simulink model "B2B_MMC"  (R2018b)
settings: Solver=ode8  StartTime=0.0  StopTime=inf  FixedStep=10e-5  RelTol=1e-3
InitFcn:
  | Cd=100e-6;
  | Csm=3.3e-3;
  | L=4e-3;
  | R=0.1;
  | m=1;
  | N=9;
  | Nminus=N-1;
  | 
  | 
  | grid.vll_rms=10e3;
  | grid.f=50;
  | w=2*pi*grid.f;
  | grid.phase=0;
  | grid.va_peak=sqrt(2/3)*grid.vll_rms;
  | 
  | vd_ref=1.05*2*sqrt(2/3)*grid.vll_rms/m; % dc link voltage in pu
  | vsp_max=0.5*m*vd_ref; %phase voltage at phi=0
  | is_max=907;
  | Smax=3*grid.va_peak*is_max/2;
  | 
  | 
  | SCR= 100;  % INPUT SCR of grid at PCC = Ssc_grid/S_rated
  | %Calculated Grid impedance parameters
  | grid.L=grid.va_peak/(w*SCR*is_max); %Calculate Lg out of SRC and neglecting Rg
  | grid.R= w*grid.L/10;        % assume Rg = 10% of Xg [ohm];
  | grid.enable=1;
  | 
  | 
  | 
  | mmc1.load_percent=100;
  | mmc1.load_pf=0.9;
  | 
  | mmc2.load_percent=100;
  | mmc2.load_pf=0.9;
  | 
  | 
  | 
  | mmc1.occ_alpha = 2000;      % INPUT Desired BW output control test converter [rad/s]
  | mmc1.occ_alpha1 = 50;       % INPUT Desired BW of the resonant integrator [rad/s]
  | mmc1.occ_alpha_f = 1000;       % INPUT Desire BW of the VFF [rad/s]
  | 
  | mmc2.occ_alpha = 2000;      % INPUT Desired BW output control test converter [rad/s]
  | mmc2.occ_alpha1 = 50;       % INPUT Desired BW of the resonant integrator [rad/s}
  | mmc2.occ_alpha_f = 1000;       % INPUT Desire BW of the VFF [rad/s
  | 
  | 
  | mmc1.ccc_enable= 1; %INPUT enable ic controller
  | mmc1.ccc_time_enable= 0; %time when circ current control kicks in [s]
  | mmc1.ccc_alpha_cr= 30;  % INPUT BW of LPF for circ current to get the reference (dc value)[rad/s]
  | mmc1.ccc_Ra        = 10;       % INPUT Proportional gain of circ current control (R << Ra < Kp)
  | mmc1.ccc_alpha2 = 200;      % INPUT BW for circulating current test converter  (alpha_c < wgrid)[rad/s]
  | 
  | mmc2.ccc_enable= 1; %INPUT enable ic controller
  | mmc2.ccc_time_enable= 0; %time when circ current control kicks in [s]
  | mmc2.ccc_alpha_cr= 30;  % INPUT BW of LPF for circ current to get the reference (dc value)[rad/s]
  | mmc2.ccc_Ra        = 10;       % INPUT Proportional gain of circ current control (R << Ra < Kp)
  | mmc2.ccc_alpha2 = 200;      % INPUT BW for circulating current test converter  (alpha_c < wgrid)[rad/s]
  | 
  | 
  | mmc1.aec_enable_W= 1; %INPUT enable arm energy controller (Wsum and Wdelta)) at time_W_ctrl
  | ... (+31 lines)
libraries: powerlib x90, powerlib_meascontrol x10, rtlab x1, rtio_opalrt_op5142ex1 x1
(part 3 of 3)

== system B2B_MMC/SM_MMC/MMC2/Control Box MMC2/Controllers/Circulating Current and Arm Energy Controller/arm energy controller /Wsum  Controller ==
  Kp_Wsum : Gain  Gain=aec.Kp_Wsum
  Mux : Mux  Inputs=2
  Mux1 : Mux  Inputs=3
  Product1 : Product
  Ripple Pass (leg a) : Subsystem
  Ripple Pass (leg b) : Subsystem
  Ripple Pass (leg c) : Subsystem
  Scope7 : Scope
  Step : Step  Time=aec.time_WsumRef_step  Before=1  After=1+aec.WsumRefStep*aec.enable_Wsum_step  SampleTime=0
  Sum6 : Sum  Inputs=+-
  "Wsum* " : Constant  Value=WsumRef
  icWsum* : Outport
  wires:
  Mux1/1 -> Sum6/2, Mux/2
  Sum6/1 -> Kp_Wsum/1
  Step/1 -> Product1/2
  Product1/1 -> Mux/1, Sum6/1
  "Wsum* "/1 -> Product1/1
  Kp_Wsum/1 -> icWsum*/1
  Mux/1 -> Scope7/1
  Ripple Pass (leg b)/1(Out1) -> Mux1/2
  Ripple Pass (leg a)/1(Out1) -> Mux1/1
  Ripple Pass (leg c)/1(Out1) -> Mux1/3
  [vc_ua] -> Ripple Pass (leg a)/1(vc_ua)
  [vc_la] -> Ripple Pass (leg a)/2(vc_la)
  [vc_lb] -> Ripple Pass (leg b)/2(vc_lb)
  [vc_ub] -> Ripple Pass (leg b)/1(vc_ub)
  [vc_lc] -> Ripple Pass (leg c)/2(vc_lc)
  [vc_uc] -> Ripple Pass (leg c)/1(vc_uc)

== system B2B_MMC/SM_MMC/MMC2/Control Box MMC2/Controllers/Circulating Current and Arm Energy Controller/ic controller/SOGI1 ==
  In : Inport
  wo : Inport  Port=2
  RST : Inport  Port=3
  Divide : Product  Inputs=**
  Divide1 : Product  Inputs=**
  Divide2 : Product  Inputs=*/
  Integrator : Integrator  ExternalReset=level
  Integrator1 : Integrator  ExternalReset=level
  Sum3 : Sum  Inputs=|+-
  Out : Outport
  wires:
  Divide1/1 -> Sum3/2
  Divide/1 -> Integrator/1
  Sum3/1 -> Divide/1
  Integrator1/1 -> Divide1/2
  In/1 -> Sum3/1
  Divide2/1 -> Out/1
  RST/1 -> Integrator/2, Integrator1/2
  wo/1 -> Divide2/2, Divide1/1, Divide/2
  Integrator/1 -> Divide2/1, Integrator1/1

== system B2B_MMC/SM_MMC/MMC2/Control Box MMC2/Controllers/Circulating Current and Arm Energy Controller/ic controller/SOGI2 ==
  In : Inport
  wo : Inport  Port=2
  RST : Inport  Port=3
  Divide : Product  Inputs=**
  Divide1 : Product  Inputs=**
  Divide2 : Product  Inputs=*/
  Integrator : Integrator  ExternalReset=level  LimitOutput=on  UpperSaturationLimit=is_max  LowerSaturationLimit=-is_max
  Integrator1 : Integrator  ExternalReset=level  LimitOutput=on  UpperSaturationLimit=is_max  LowerSaturationLimit=-is_max
  Sum3 : Sum  Inputs=|+-
  Out : Outport
  wires:
  Integrator/1 -> Divide2/1, Integrator1/1
  wo/1 -> Divide/2, Divide1/1, Divide2/2
  RST/1 -> Integrator/2, Integrator1/2
  Divide2/1 -> Out/1
  In/1 -> Sum3/1
  Integrator1/1 -> Divide1/2
  Sum3/1 -> Divide/1
  Divide/1 -> Integrator/1
  Divide1/1 -> Sum3/2

== system B2B_MMC/SM_MMC/MMC2/Control Box MMC2/Controllers/PR Output Current Controller/Subsystem/PR ==
  note: SOGI continuous=sw/(s2+w2)
  In : Inport
  w0 : Inport  Port=2
  Gain3 : Gain  Gain=occ.K1
  SOGI : Subsystem
  Step : Step  Time=0.0001  Before=1  After=0  SampleTime=0
  Out : Outport
  wires:
  Gain3/1 -> Out/1
  In/1 -> SOGI/1(In)
  w0/1 -> SOGI/2(wo)
  [occRST] -> SOGI/3(RST)
  SOGI/1(Out) -> Gain3/1
  Step/1 -> [occRST]

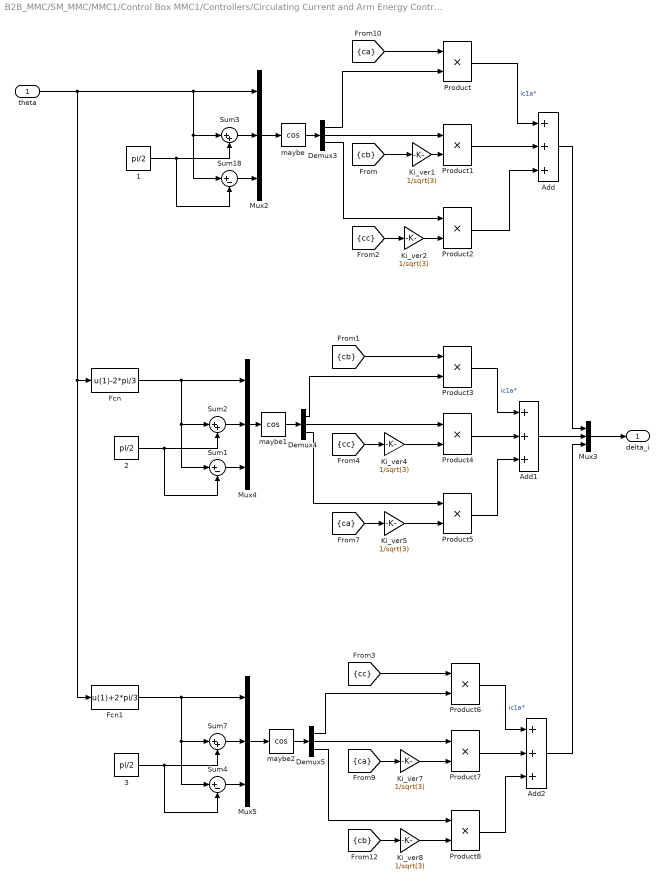
== system B2B_MMC/SM_MMC/MMC1/Control Box MMC1/Controllers/Circulating Current and Arm Energy Controller/arm energy controller /Wdelta  Controller/correction ==
  theta : Inport
  "  1" : Constant  Value=pi/2
  "  2" : Constant  Value=pi/2
  "  3" : Constant  Value=pi/2
  Add : Sum  Inputs=+++
  Add1 : Sum  Inputs=+++
  Add2 : Sum  Inputs=+++
  Demux3 : Demux  Outputs=3
  Demux4 : Demux  Outputs=3
  Demux5 : Demux  Outputs=3
  Fcn : Fcn  Expr=u(1)-2*pi/3
  Fcn1 : Fcn  Expr=u(1)+2*pi/3
  Ki_ver{1..2,4..5,7..8} (6 alike) : Gain  Gain=1/sqrt(3)
  Mux{2..5} (4 alike) : Mux  Inputs=3
  Product{,1..8} (9 alike) : Product
  Sum1 : Sum  Inputs=|+-
  Sum18 : Sum  Inputs=|+-
  Sum2 : Sum  Inputs=|++
  Sum3 : Sum  Inputs=|++
  Sum4 : Sum  Inputs=|+-
  Sum7 : Sum  Inputs=|++
  maybe : Trigonometry  Operator=cos
  maybe1 : Trigonometry  Operator=cos
  maybe2 : Trigonometry  Operator=cos
  delta_i : Outport
  wires:
  Demux4/2 -> Product4/1
  Demux4/3 -> Product5/1
  [ca] -> Product/1
  [ca] -> Ki_ver7/1
  Sum4/1 -> Mux5/3
  Demux4/1 -> Product3/2
  Mux4/1 -> maybe1/1
  Add/1 -> Mux3/1
  Sum3/1 -> Mux2/2
  Ki_ver7/1 -> Product7/2
  Sum7/1 -> Mux5/2
  [cb] -> Ki_ver1/1
  Product1/1 -> Add/2
  Add2/1 -> Mux3/3
  Product5/1 -> Add1/3
  Product8/1 -> Add2/3
  Product3/1 -> Add1/1  "ic1a*"
  Sum18/1 -> Mux2/3
  Add1/1 -> Mux3/2
  "  2"/1 -> Sum1/2, Sum2/2
  Mux5/1 -> maybe2/1
  Demux5/3 -> Product8/1
  Ki_ver4/1 -> Product4/2
  Demux3/1 -> Product/2
  theta/1 -> Mux2/1, Sum3/1, Sum18/1, Fcn/1, Fcn1/1
  maybe1/1 -> Demux4/1
  [cc] -> Ki_ver4/1
  Product7/1 -> Add2/2
  maybe2/1 -> Demux5/1
  Sum2/1 -> Mux4/2
  Demux5/2 -> Product7/1
  Ki_ver5/1 -> Product5/2
  Ki_ver1/1 -> Product1/2
  [cb] -> Product3/1
  Demux5/1 -> Product6/2
  Product/1 -> Add/1  "ic1a*"
  [cb] -> Ki_ver8/1
  maybe/1 -> Demux3/1
  "  3"/1 -> Sum7/2, Sum4/2
  Sum1/1 -> Mux4/3
  Product4/1 -> Add1/2
  Ki_ver2/1 -> Product2/2
  Product2/1 -> Add/3
  [cc] -> Ki_ver2/1
  Ki_ver8/1 -> Product8/2
  "  1"/1 -> Sum3/2, Sum18/2
  Demux3/2 -> Product1/1
  Fcn1/1 -> Mux5/1, Sum7/1, Sum4/1
  Demux3/3 -> Product2/1
  Fcn/1 -> Sum1/1, Sum2/1, Mux4/1
  [ca] -> Ki_ver5/1
  Product6/1 -> Add2/1  "ic1a*"
  Mux2/1 -> maybe/1
  Mux3/1 -> delta_i/1
  [cc] -> Product6/1

== system B2B_MMC/SM_MMC/MMC1/Control Box MMC1/Controllers/Circulating Current and Arm Energy Controller/arm energy controller /Wdelta  Controller/ripple pass (leg a) ==
  vc_ua : Inport
  vc_la : Inport  Port=2
  BandStop @100Hz_10kHz : TransferFcn  Numerator=[1 0 2*w*2*w]  Denominator=[1 2*2*w 2*w*2*w]
  BandStop @50Hz_10kHz1 : TransferFcn  Numerator=[1 0 w*w]  Denominator=[1 2*w w*w]
  Gain : Gain  Gain=Csm/2/N
  Math Function : Math  Operator=square  SaturateOnIntegerOverflow=on
  Math Function1 : Math  Operator=square  SaturateOnIntegerOverflow=on
  Sum : Sum  Inputs=|+-
  Sum of Elements : Sum  Inputs=+
  Sum of Elements1 : Sum  Inputs=+
  Out1 : Outport
  wires:
  BandStop @100Hz_10kHz/1 -> Out1/1
  Math Function1/1 -> Sum/2
  Gain/1 -> BandStop @50Hz_10kHz1/1
  Math Function/1 -> Sum/1
  BandStop @50Hz_10kHz1/1 -> BandStop @100Hz_10kHz/1
  Sum/1 -> Gain/1
  Sum of Elements/1 -> Math Function/1
  vc_ua/1 -> Sum of Elements/1
  Sum of Elements1/1 -> Math Function1/1
  vc_la/1 -> Sum of Elements1/1

== system B2B_MMC/SM_MMC/MMC1/Control Box MMC1/Controllers/Circulating Current and Arm Energy Controller/arm energy controller /Wdelta  Controller/ripple pass (leg b) ==
  vc_ub : Inport
  vc_lb : Inport  Port=2
  BandStop @100Hz_10kHz : TransferFcn  Numerator=[1 0 2*w*2*w]  Denominator=[1 2*2*w 2*w*2*w]
  BandStop @50Hz_10kHz1 : TransferFcn  Numerator=[1 0 w*w]  Denominator=[1 2*w w*w]
  Gain : Gain  Gain=Csm/2/N
  Math Function : Math  Operator=square  SaturateOnIntegerOverflow=on
  Math Function1 : Math  Operator=square  SaturateOnIntegerOverflow=on
  Sum : Sum  Inputs=|+-
  Sum of Elements : Sum  Inputs=+
  Sum of Elements1 : Sum  Inputs=+
  Out1 : Outport
  wires:
  BandStop @100Hz_10kHz/1 -> Out1/1
  Math Function1/1 -> Sum/2
  Gain/1 -> BandStop @50Hz_10kHz1/1
  Math Function/1 -> Sum/1
  BandStop @50Hz_10kHz1/1 -> BandStop @100Hz_10kHz/1
  Sum/1 -> Gain/1
  Sum of Elements/1 -> Math Function/1
  vc_ub/1 -> Sum of Elements/1
  Sum of Elements1/1 -> Math Function1/1
  vc_lb/1 -> Sum of Elements1/1

== system B2B_MMC/SM_MMC/MMC1/Control Box MMC1/Controllers/Circulating Current and Arm Energy Controller/arm energy controller /Wdelta  Controller/ripple pass (leg c) ==
  vc_uc : Inport
  vc_lc : Inport  Port=2
  BandStop @100Hz_10kHz : TransferFcn  Numerator=[1 0 2*w*2*w]  Denominator=[1 2*2*w 2*w*2*w]
  BandStop @50Hz_10kHz1 : TransferFcn  Numerator=[1 0 w*w]  Denominator=[1 2*w w*w]
  Gain : Gain  Gain=Csm/2/N
  Math Function : Math  Operator=square  SaturateOnIntegerOverflow=on
  Math Function1 : Math  Operator=square  SaturateOnIntegerOverflow=on
  Sum : Sum  Inputs=|+-
  Sum of Elements : Sum  Inputs=+
  Sum of Elements1 : Sum  Inputs=+
  Out1 : Outport
  wires:
  BandStop @100Hz_10kHz/1 -> Out1/1
  Math Function1/1 -> Sum/2
  Gain/1 -> BandStop @50Hz_10kHz1/1
  Math Function/1 -> Sum/1
  BandStop @50Hz_10kHz1/1 -> BandStop @100Hz_10kHz/1
  Sum/1 -> Gain/1
  Sum of Elements/1 -> Math Function/1
  vc_uc/1 -> Sum of Elements/1
  Sum of Elements1/1 -> Math Function1/1
  vc_lc/1 -> Sum of Elements1/1

== system B2B_MMC/SM_MMC/MMC1/Control Box MMC1/Controllers/Circulating Current and Arm Energy Controller/arm energy controller /Wsum  Controller/Ripple Pass (leg a) ==
  vc_ua : Inport
  vc_la : Inport  Port=2
  BandStop @100Hz_10kHz1 : TransferFcn  Numerator=[1 0 2*w*2*w]  Denominator=[1 2*2*w 2*w*2*w]
  BandStop @50Hz_10kHz1 : TransferFcn  Numerator=[1 0 w*w]  Denominator=[1 2*w w*w]
  Gain : Gain  Gain=Csm/(2*N)
  Math Function : Math  Operator=square  SaturateOnIntegerOverflow=on
  Math Function1 : Math  Operator=square  SaturateOnIntegerOverflow=on
  Sum : Sum  Inputs=|++
  Sum of Elements : Sum  Inputs=+
  Sum of Elements1 : Sum  Inputs=+
  Out1 : Outport
  wires:
  BandStop @50Hz_10kHz1/1 -> BandStop @100Hz_10kHz1/1
  Math Function/1 -> Sum/1
  Sum/1 -> Gain/1
  Math Function1/1 -> Sum/2
  Gain/1 -> BandStop @50Hz_10kHz1/1
  BandStop @100Hz_10kHz1/1 -> Out1/1
  vc_ua/1 -> Sum of Elements/1
  Sum of Elements/1 -> Math Function/1
  vc_la/1 -> Sum of Elements1/1
  Sum of Elements1/1 -> Math Function1/1

== system B2B_MMC/SM_MMC/MMC1/Control Box MMC1/Controllers/Circulating Current and Arm Energy Controller/arm energy controller /Wsum  Controller/Ripple Pass (leg b) ==
  vc_ub : Inport
  vc_lb : Inport  Port=2
  BandStop @100Hz_10kHz1 : TransferFcn  Numerator=[1 0 2*w*2*w]  Denominator=[1 2*2*w 2*w*2*w]
  BandStop @50Hz_10kHz1 : TransferFcn  Numerator=[1 0 w*w]  Denominator=[1 2*w w*w]
  Gain : Gain  Gain=Csm/(2*N)
  Math Function : Math  Operator=square  SaturateOnIntegerOverflow=on
  Math Function1 : Math  Operator=square  SaturateOnIntegerOverflow=on
  Sum : Sum  Inputs=|++
  Sum of Elements : Sum  Inputs=+
  Sum of Elements1 : Sum  Inputs=+
  Out1 : Outport
  wires:
  BandStop @50Hz_10kHz1/1 -> BandStop @100Hz_10kHz1/1
  Math Function/1 -> Sum/1
  Sum/1 -> Gain/1
  Math Function1/1 -> Sum/2
  Gain/1 -> BandStop @50Hz_10kHz1/1
  BandStop @100Hz_10kHz1/1 -> Out1/1
  Sum of Elements/1 -> Math Function/1
  vc_ub/1 -> Sum of Elements/1
  Sum of Elements1/1 -> Math Function1/1
  vc_lb/1 -> Sum of Elements1/1

== system B2B_MMC/SM_MMC/MMC1/Control Box MMC1/Controllers/Circulating Current and Arm Energy Controller/arm energy controller /Wsum  Controller/Ripple Pass (leg c) ==
  vc_uc : Inport
  vc_lc : Inport  Port=2
  BandStop @100Hz_10kHz1 : TransferFcn  Numerator=[1 0 2*w*2*w]  Denominator=[1 2*2*w 2*w*2*w]
  BandStop @50Hz_10kHz1 : TransferFcn  Numerator=[1 0 w*w]  Denominator=[1 2*w w*w]
  Gain : Gain  Gain=Csm/(2*N)
  Math Function : Math  Operator=square  SaturateOnIntegerOverflow=on
  Math Function1 : Math  Operator=square  SaturateOnIntegerOverflow=on
  Sum : Sum  Inputs=|++
  Sum of Elements : Sum  Inputs=+
  Sum of Elements1 : Sum  Inputs=+
  Out1 : Outport
  wires:
  BandStop @50Hz_10kHz1/1 -> BandStop @100Hz_10kHz1/1
  Math Function/1 -> Sum/1
  Sum/1 -> Gain/1
  Math Function1/1 -> Sum/2
  Gain/1 -> BandStop @50Hz_10kHz1/1
  BandStop @100Hz_10kHz1/1 -> Out1/1
  Sum of Elements/1 -> Math Function/1
  vc_uc/1 -> Sum of Elements/1
  Sum of Elements1/1 -> Math Function1/1
  vc_lc/1 -> Sum of Elements1/1

== system B2B_MMC/SM_MMC/MMC1/Control Box MMC1/Controllers/PR Output Current Controller/Subsystem/PR/SOGI ==
  In : Inport
  wo : Inport  Port=2
  RST : Inport  Port=3
  Divide : Product  Inputs=**
  Divide1 : Product  Inputs=**
  Divide2 : Product  Inputs=*/
  Integrator : Integrator  ExternalReset=level
  Integrator2 : Integrator  ExternalReset=level
  Sum3 : Sum  Inputs=|+-
  Out : Outport
  wires:
  Divide1/1 -> Sum3/2
  Divide/1 -> Integrator/1
  Sum3/1 -> Divide/1
  Integrator2/1 -> Divide1/2
  In/1 -> Sum3/1
  Divide2/1 -> Out/1
  wo/1 -> Divide2/2, Divide1/1, Divide/2
  RST/1 -> Integrator2/2, Integrator/2
  Integrator/1 -> Integrator2/1, Divide2/1

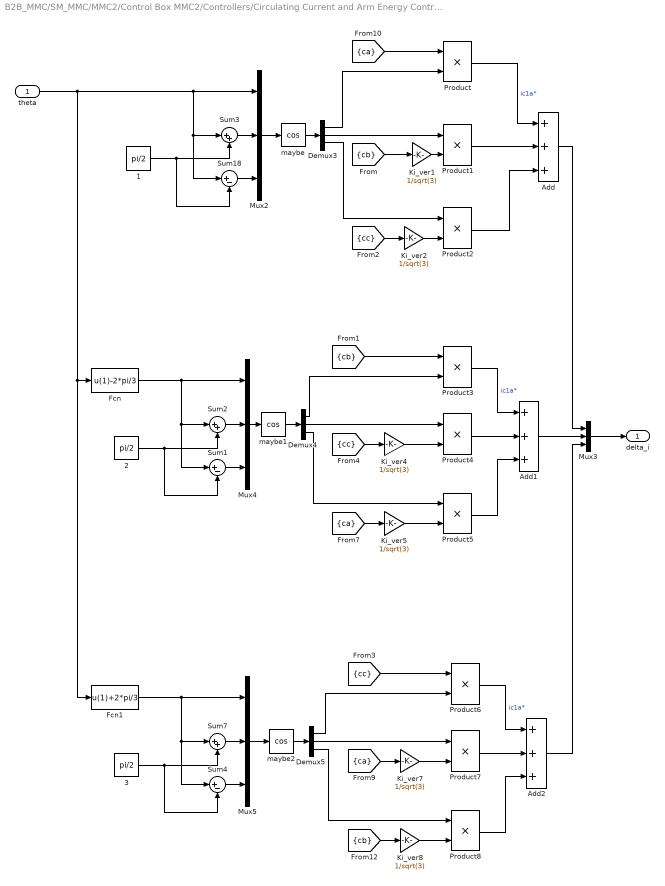
== system B2B_MMC/SM_MMC/MMC2/Control Box MMC2/Controllers/Circulating Current and Arm Energy Controller/arm energy controller /Wdelta  Controller/correction ==
  theta : Inport
  "  1" : Constant  Value=pi/2
  "  2" : Constant  Value=pi/2
  "  3" : Constant  Value=pi/2
  Add : Sum  Inputs=+++
  Add1 : Sum  Inputs=+++
  Add2 : Sum  Inputs=+++
  Demux3 : Demux  Outputs=3
  Demux4 : Demux  Outputs=3
  Demux5 : Demux  Outputs=3
  Fcn : Fcn  Expr=u(1)-2*pi/3
  Fcn1 : Fcn  Expr=u(1)+2*pi/3
  Ki_ver{1..2,4..5,7..8} (6 alike) : Gain  Gain=1/sqrt(3)
  Mux{2..5} (4 alike) : Mux  Inputs=3
  Product{,1..8} (9 alike) : Product
  Sum1 : Sum  Inputs=|+-
  Sum18 : Sum  Inputs=|+-
  Sum2 : Sum  Inputs=|++
  Sum3 : Sum  Inputs=|++
  Sum4 : Sum  Inputs=|+-
  Sum7 : Sum  Inputs=|++
  maybe : Trigonometry  Operator=cos
  maybe1 : Trigonometry  Operator=cos
  maybe2 : Trigonometry  Operator=cos
  delta_i : Outport
  wires:
  Demux4/2 -> Product4/1
  Demux4/3 -> Product5/1
  [ca] -> Product/1
  [ca] -> Ki_ver7/1
  Sum4/1 -> Mux5/3
  Demux4/1 -> Product3/2
  Mux4/1 -> maybe1/1
  Add/1 -> Mux3/1
  Sum3/1 -> Mux2/2
  Ki_ver7/1 -> Product7/2
  Sum7/1 -> Mux5/2
  [cb] -> Ki_ver1/1
  Product1/1 -> Add/2
  Add2/1 -> Mux3/3
  Product5/1 -> Add1/3
  Product8/1 -> Add2/3
  Product3/1 -> Add1/1  "ic1a*"
  Sum18/1 -> Mux2/3
  Add1/1 -> Mux3/2
  "  2"/1 -> Sum1/2, Sum2/2
  Mux5/1 -> maybe2/1
  Demux5/3 -> Product8/1
  Ki_ver4/1 -> Product4/2
  Demux3/1 -> Product/2
  theta/1 -> Mux2/1, Sum3/1, Sum18/1, Fcn/1, Fcn1/1
  maybe1/1 -> Demux4/1
  [cc] -> Ki_ver4/1
  Product7/1 -> Add2/2
  maybe2/1 -> Demux5/1
  Sum2/1 -> Mux4/2
  Demux5/2 -> Product7/1
  Ki_ver5/1 -> Product5/2
  Ki_ver1/1 -> Product1/2
  [cb] -> Product3/1
  Demux5/1 -> Product6/2
  Product/1 -> Add/1  "ic1a*"
  [cb] -> Ki_ver8/1
  maybe/1 -> Demux3/1
  "  3"/1 -> Sum7/2, Sum4/2
  Sum1/1 -> Mux4/3
  Product4/1 -> Add1/2
  Ki_ver2/1 -> Product2/2
  Product2/1 -> Add/3
  [cc] -> Ki_ver2/1
  Ki_ver8/1 -> Product8/2
  "  1"/1 -> Sum3/2, Sum18/2
  Demux3/2 -> Product1/1
  Fcn1/1 -> Mux5/1, Sum7/1, Sum4/1
  Demux3/3 -> Product2/1
  Fcn/1 -> Sum1/1, Sum2/1, Mux4/1
  [ca] -> Ki_ver5/1
  Product6/1 -> Add2/1  "ic1a*"
  Mux2/1 -> maybe/1
  Mux3/1 -> delta_i/1
  [cc] -> Product6/1

== system B2B_MMC/SM_MMC/MMC2/Control Box MMC2/Controllers/Circulating Current and Arm Energy Controller/arm energy controller /Wdelta  Controller/ripple pass (leg a) ==
  vc_ua : Inport
  vc_la : Inport  Port=2
  BandStop @100Hz_10kHz : TransferFcn  Numerator=[1 0 2*w*2*w]  Denominator=[1 2*2*w 2*w*2*w]
  BandStop @50Hz_10kHz1 : TransferFcn  Numerator=[1 0 w*w]  Denominator=[1 2*w w*w]
  Gain : Gain  Gain=Csm/2/N
  Math Function : Math  Operator=square  SaturateOnIntegerOverflow=on
  Math Function1 : Math  Operator=square  SaturateOnIntegerOverflow=on
  Sum : Sum  Inputs=|+-
  Sum of Elements : Sum  Inputs=+
  Sum of Elements1 : Sum  Inputs=+
  Out1 : Outport
  wires:
  BandStop @100Hz_10kHz/1 -> Out1/1
  Math Function1/1 -> Sum/2
  Gain/1 -> BandStop @50Hz_10kHz1/1
  Math Function/1 -> Sum/1
  BandStop @50Hz_10kHz1/1 -> BandStop @100Hz_10kHz/1
  Sum/1 -> Gain/1
  Sum of Elements/1 -> Math Function/1
  vc_ua/1 -> Sum of Elements/1
  Sum of Elements1/1 -> Math Function1/1
  vc_la/1 -> Sum of Elements1/1

== system B2B_MMC/SM_MMC/MMC2/Control Box MMC2/Controllers/Circulating Current and Arm Energy Controller/arm energy controller /Wdelta  Controller/ripple pass (leg b) ==
  vc_ub : Inport
  vc_lb : Inport  Port=2
  BandStop @100Hz_10kHz : TransferFcn  Numerator=[1 0 2*w*2*w]  Denominator=[1 2*2*w 2*w*2*w]
  BandStop @50Hz_10kHz1 : TransferFcn  Numerator=[1 0 w*w]  Denominator=[1 2*w w*w]
  Gain : Gain  Gain=Csm/2/N
  Math Function : Math  Operator=square  SaturateOnIntegerOverflow=on
  Math Function1 : Math  Operator=square  SaturateOnIntegerOverflow=on
  Sum : Sum  Inputs=|+-
  Sum of Elements : Sum  Inputs=+
  Sum of Elements1 : Sum  Inputs=+
  Out1 : Outport
  wires:
  BandStop @100Hz_10kHz/1 -> Out1/1
  Math Function1/1 -> Sum/2
  Gain/1 -> BandStop @50Hz_10kHz1/1
  Math Function/1 -> Sum/1
  BandStop @50Hz_10kHz1/1 -> BandStop @100Hz_10kHz/1
  Sum/1 -> Gain/1
  Sum of Elements/1 -> Math Function/1
  vc_ub/1 -> Sum of Elements/1
  Sum of Elements1/1 -> Math Function1/1
  vc_lb/1 -> Sum of Elements1/1

== system B2B_MMC/SM_MMC/MMC2/Control Box MMC2/Controllers/Circulating Current and Arm Energy Controller/arm energy controller /Wdelta  Controller/ripple pass (leg c) ==
  vc_uc : Inport
  vc_lc : Inport  Port=2
  BandStop @100Hz_10kHz : TransferFcn  Numerator=[1 0 2*w*2*w]  Denominator=[1 2*2*w 2*w*2*w]
  BandStop @50Hz_10kHz1 : TransferFcn  Numerator=[1 0 w*w]  Denominator=[1 2*w w*w]
  Gain : Gain  Gain=Csm/2/N
  Math Function : Math  Operator=square  SaturateOnIntegerOverflow=on
  Math Function1 : Math  Operator=square  SaturateOnIntegerOverflow=on
  Sum : Sum  Inputs=|+-
  Sum of Elements : Sum  Inputs=+
  Sum of Elements1 : Sum  Inputs=+
  Out1 : Outport
  wires:
  BandStop @100Hz_10kHz/1 -> Out1/1
  Math Function1/1 -> Sum/2
  Gain/1 -> BandStop @50Hz_10kHz1/1
  Math Function/1 -> Sum/1
  BandStop @50Hz_10kHz1/1 -> BandStop @100Hz_10kHz/1
  Sum/1 -> Gain/1
  Sum of Elements/1 -> Math Function/1
  vc_uc/1 -> Sum of Elements/1
  Sum of Elements1/1 -> Math Function1/1
  vc_lc/1 -> Sum of Elements1/1

== system B2B_MMC/SM_MMC/MMC2/Control Box MMC2/Controllers/Circulating Current and Arm Energy Controller/arm energy controller /Wsum  Controller/Ripple Pass (leg a) ==
  vc_ua : Inport
  vc_la : Inport  Port=2
  BandStop @100Hz_10kHz1 : TransferFcn  Numerator=[1 0 2*w*2*w]  Denominator=[1 2*2*w 2*w*2*w]
  BandStop @50Hz_10kHz1 : TransferFcn  Numerator=[1 0 w*w]  Denominator=[1 2*w w*w]
  Gain : Gain  Gain=Csm/(2*N)
  Math Function : Math  Operator=square  SaturateOnIntegerOverflow=on
  Math Function1 : Math  Operator=square  SaturateOnIntegerOverflow=on
  Sum : Sum  Inputs=|++
  Sum of Elements : Sum  Inputs=+
  Sum of Elements1 : Sum  Inputs=+
  Out1 : Outport
  wires:
  BandStop @50Hz_10kHz1/1 -> BandStop @100Hz_10kHz1/1
  Math Function/1 -> Sum/1
  Sum/1 -> Gain/1
  Math Function1/1 -> Sum/2
  Gain/1 -> BandStop @50Hz_10kHz1/1
  BandStop @100Hz_10kHz1/1 -> Out1/1
  vc_ua/1 -> Sum of Elements/1
  Sum of Elements/1 -> Math Function/1
  vc_la/1 -> Sum of Elements1/1
  Sum of Elements1/1 -> Math Function1/1

== system B2B_MMC/SM_MMC/MMC2/Control Box MMC2/Controllers/Circulating Current and Arm Energy Controller/arm energy controller /Wsum  Controller/Ripple Pass (leg b) ==
  vc_ub : Inport
  vc_lb : Inport  Port=2
  BandStop @100Hz_10kHz1 : TransferFcn  Numerator=[1 0 2*w*2*w]  Denominator=[1 2*2*w 2*w*2*w]
  BandStop @50Hz_10kHz1 : TransferFcn  Numerator=[1 0 w*w]  Denominator=[1 2*w w*w]
  Gain : Gain  Gain=Csm/(2*N)
  Math Function : Math  Operator=square  SaturateOnIntegerOverflow=on
  Math Function1 : Math  Operator=square  SaturateOnIntegerOverflow=on
  Sum : Sum  Inputs=|++
  Sum of Elements : Sum  Inputs=+
  Sum of Elements1 : Sum  Inputs=+
  Out1 : Outport
  wires:
  BandStop @50Hz_10kHz1/1 -> BandStop @100Hz_10kHz1/1
  Math Function/1 -> Sum/1
  Sum/1 -> Gain/1
  Math Function1/1 -> Sum/2
  Gain/1 -> BandStop @50Hz_10kHz1/1
  BandStop @100Hz_10kHz1/1 -> Out1/1
  Sum of Elements/1 -> Math Function/1
  vc_ub/1 -> Sum of Elements/1
  Sum of Elements1/1 -> Math Function1/1
  vc_lb/1 -> Sum of Elements1/1

== system B2B_MMC/SM_MMC/MMC2/Control Box MMC2/Controllers/Circulating Current and Arm Energy Controller/arm energy controller /Wsum  Controller/Ripple Pass (leg c) ==
  vc_uc : Inport
  vc_lc : Inport  Port=2
  BandStop @100Hz_10kHz1 : TransferFcn  Numerator=[1 0 2*w*2*w]  Denominator=[1 2*2*w 2*w*2*w]
  BandStop @50Hz_10kHz1 : TransferFcn  Numerator=[1 0 w*w]  Denominator=[1 2*w w*w]
  Gain : Gain  Gain=Csm/(2*N)
  Math Function : Math  Operator=square  SaturateOnIntegerOverflow=on
  Math Function1 : Math  Operator=square  SaturateOnIntegerOverflow=on
  Sum : Sum  Inputs=|++
  Sum of Elements : Sum  Inputs=+
  Sum of Elements1 : Sum  Inputs=+
  Out1 : Outport
  wires:
  BandStop @50Hz_10kHz1/1 -> BandStop @100Hz_10kHz1/1
  Math Function/1 -> Sum/1
  Sum/1 -> Gain/1
  Math Function1/1 -> Sum/2
  Gain/1 -> BandStop @50Hz_10kHz1/1
  BandStop @100Hz_10kHz1/1 -> Out1/1
  Sum of Elements/1 -> Math Function/1
  vc_uc/1 -> Sum of Elements/1
  Sum of Elements1/1 -> Math Function1/1
  vc_lc/1 -> Sum of Elements1/1

== system B2B_MMC/SM_MMC/MMC2/Control Box MMC2/Controllers/PR Output Current Controller/Subsystem/PR/SOGI ==
  In : Inport
  wo : Inport  Port=2
  RST : Inport  Port=3
  Divide : Product  Inputs=**
  Divide1 : Product  Inputs=**
  Divide2 : Product  Inputs=*/
  Integrator : Integrator  ExternalReset=level
  Integrator2 : Integrator  ExternalReset=level
  Sum3 : Sum  Inputs=|+-
  Out : Outport
  wires:
  Divide1/1 -> Sum3/2
  Divide/1 -> Integrator/1
  Sum3/1 -> Divide/1
  Integrator2/1 -> Divide1/2
  In/1 -> Sum3/1
  Divide2/1 -> Out/1
  wo/1 -> Divide2/2, Divide1/1, Divide/2
  RST/1 -> Integrator2/2, Integrator/2
  Integrator/1 -> Integrator2/1, Divide2/1
